simulink model "QuaterCarSuspensionPIDmodel"  (R2025b)
settings: Solver=VariableStepAuto  StartTime=0.0  StopTime=10.0  RelTol=1e-3
values from neighbouring files (symbols this model uses):
  c = 100    [initialize_LF.m]    (also in initialize_PID.m = 300)
  G = 10000    [initialize_PID.m]
  k = 10000    [initialize_LF.m]    (also in initialize_PID.m)
  kd = 0.2    [initialize_PID.m]
  ki = 0.5    [initialize_PID.m]
  kp = 10    [initialize_PID.m]
  m = 200    [initialize_LF.m]    (also in initialize_PID.m = 300)
settings Model: Creator=kanch  LastModifiedBy=kanch
settings DataIOCC: ExternalInput=inputDataStructure  LoadExternalInput=on

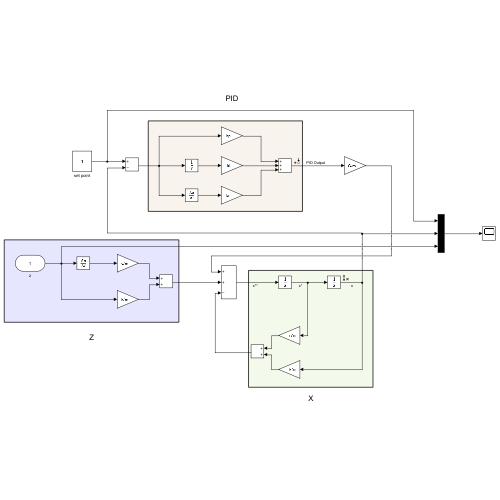
[thumbnail: Simulink's stored preview of the top-level diagram]
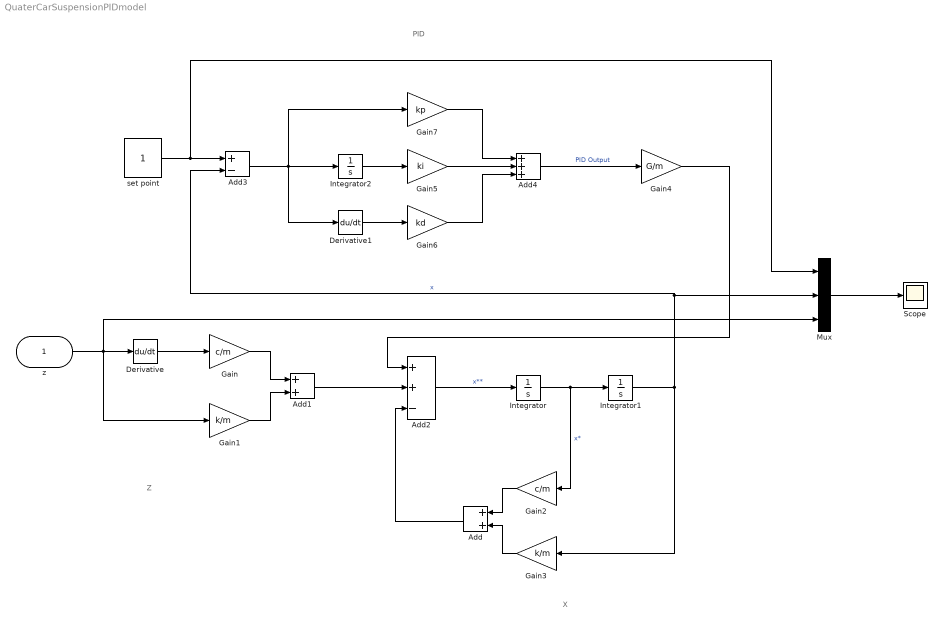
== system QuaterCarSuspensionPIDmodel ==
  note: Z
  note: X
  note: PID
  z : Inport
  Add : Sum
  Add1 : Sum
  Add2 : Sum  Inputs=++-
  Add3 : Sum  Inputs=+-
  Add4 : Sum  Inputs=+++
  Derivative : Derivative
  Derivative1 : Derivative
  Gain : Gain  Gain=c/m
  Gain1 : Gain  Gain=k/m
  Gain2 : Gain  Gain=c/m
  Gain3 : Gain  Gain=k/m
  Gain4 : Gain  Gain=G/m
  Gain5 : Gain  Gain=ki
  Gain6 : Gain  Gain=kd
  Gain7 : Gain  Gain=kp
  Integrator : Integrator
  Integrator1 : Integrator
  Integrator2 : Integrator
  Mux : Mux  Inputs=3
  Scope : Scope
      settings: ActiveDisplayYMinimum=-2.1876786977184919  ActiveDisplayYMaximum=2.7416007571594685
  set point : Constant
  wires:
  z/1 -> Mux/3, Gain1/1, Derivative/1
  Derivative/1 -> Gain/1
  Add2/1 -> Integrator/1  "x**"
  Integrator/1 -> Gain2/1, Integrator1/1  "x*"
  Integrator1/1 -> Gain3/1, Mux/2, Add3/2  "x"
  Gain2/1 -> Add/1
  Gain3/1 -> Add/2
  Gain/1 -> Add1/1
  Gain1/1 -> Add1/2
  Add/1 -> Add2/3
  Add1/1 -> Add2/2
  set point/1 -> Add3/1, Mux/1
  Add3/1 -> Derivative1/1, Integrator2/1, Gain7/1
  Integrator2/1 -> Gain5/1
  Derivative1/1 -> Gain6/1
  Gain4/1 -> Add2/1
  Add4/1 -> Gain4/1  "PID Output"
  Gain5/1 -> Add4/2
  Gain6/1 -> Add4/3
  Gain7/1 -> Add4/1
  Mux/1 -> Scope/1
